simulink model "MATMPC_SIMULINK_R2022b"  (R2022b)
settings: Solver=ode4  StartTime=0.0  StopTime=10  RelTol=1e-3
values from neighbouring files (symbols this model uses):
  lb = 0    [Initialization_Simulink.m]
  lbu = -inf(nu,1)    [InitData.m]    (also in Initialization_Simulink.m = repmat(lbu,1,N))
  lbx = 0    [Initialization_Simulink.m]
  para = repmat(para0,1,N+1)    [InitData.m]    (also in Initialization_Simulink.m)
  Ts = settings.Ts_st    [Initialization_Simulink.m]    (also in Simulation.m)
  ub = 0    [Initialization_Simulink.m]
  ubu = inf(nu,1)    [InitData.m]    (also in Initialization_Simulink.m = repmat(ubu,1,N))
  ubx = 0    [Initialization_Simulink.m]
  W = repmat([Qp Qrpy Qq Qv Qomega Qdu]',1,N)    [Initialization_Simulink.m]
  WN = [Qp Qrpy Qq Qv Qomega]'    [Initialization_Simulink.m]
  x0 = [ ... (first row only)    [Initialization_Simulink.m]
  z0 = 0    [Initialization_Simulink.m]
undefined symbols (not defined in the file or in its folder): opt, settings
libraries: sharedtransform x1, simulink_extras x1, sharedTrackingLibrary x1
settings Model: Creator=chen  LastModifiedBy=beniamino
settings SolverCC: AlgebraicLoopSolver=TrustRegion
settings DataIOCC: ReturnWorkspaceOutputs=off
settings DebuggingCC: UnconnectedInputMsg=warning  UnconnectedOutputMsg=warning  UnconnectedLineMsg=warning  SFMachineParentedDataDiag=warning  ArithmeticOperatorsInVariantConditions=warning
settings ModelReferenceCC: EnableRefExpFcnMdlSchedulingChecks=on
settings SFSimCC: SimUseLocalCustomCode=off  CustomCodeUndefinedFunction=UseInterfaceOnly
settings RTWCC: RTWUseLocalCustomCode=off  CheckMdlBeforeBuild=Error

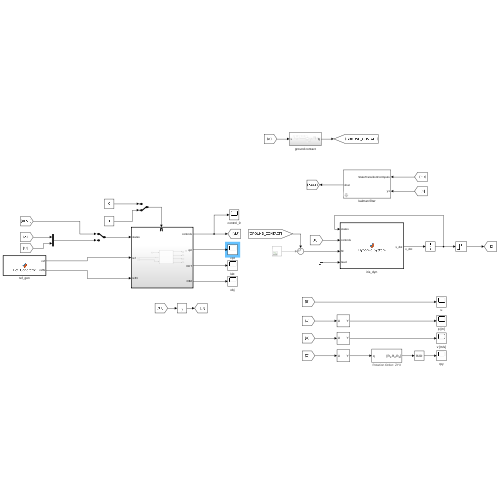
[thumbnail: Simulink's stored preview of the top-level diagram]
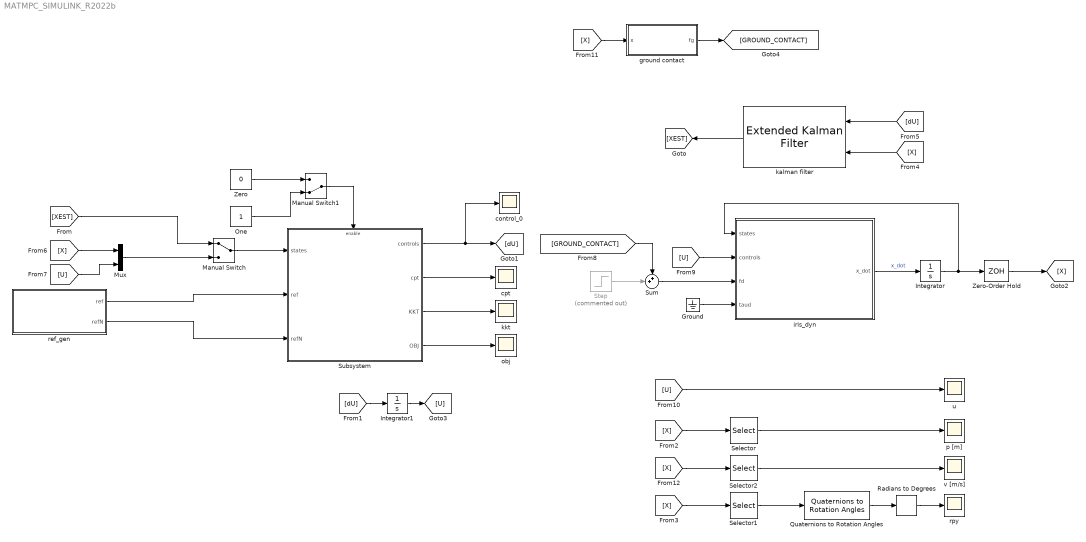
== system MATMPC_SIMULINK_R2022b ==
  Ground : Ground
  Integrator : Integrator  InitialCondition=x0(1:13)
  Integrator1 : Integrator  InitialCondition=[0.5 0.5 0.5 0.5]
  Manual Switch : ManualSwitch
  Manual Switch1 : ManualSwitch  CurrentSetting=0
  Mux : Mux  Inputs=2
  One : Constant  OutDataTypeStr=Inherit: Inherit via back propagation
  Quaternions to Rotation Angles : sharedtransform/Quaternions to Rotation Angles  rotationOrder=ZYX  aMode=aMode
  Radians to Degrees : simulink_extras/Transformations/Radians to Degrees
  Selector : Selector  InputPortWidth=13  IndexOptions=Index vector (dialog)  Indices=[1 2 3]  OutputSizes=1
  Selector1 : Selector  InputPortWidth=13  IndexOptions=Index vector (dialog)  Indices=4:7  OutputSizes=1
  Selector2 : Selector  InputPortWidth=13  IndexOptions=Index vector (dialog)  Indices=8:10  OutputSizes=1
  Step : Step  Commented=on  Time=5  Before=[0 0 0]  After=[1 0 0]  SampleTime=Ts
  Subsystem : Subsystem
  Sum : Sum  Inputs=++|
  Zero : Constant  Value=0  OutDataTypeStr=Inherit: Inherit via back propagation
  Zero-Order Hold : ZeroOrderHold  SampleTime=Ts
  control_0 : Scope
  cpt : Scope
  ground contact : Subsystem
  iris_dyn : MATLAB Function  TreatAsAtomicUnit=on
  kalman filter : sharedTrackingLibrary/Extended Kalman Filter  StateTransitionFcn=irisStateTransitionFcn  HasStateTransitionJacobianFcn=off  HasAdditiveProcessNoise=Additive  ProcessNoise=Q  HasTimeVaryingProcessNoise=off  HasStateTransitionFcnExtraArgument=1  InitialState=x0  InitialStateCovariance=Q0  MeasurementFcn1=irisMeasurementFcn  HasMeasurementJacobianFcn1=off  HasMeasurementEnablePort1=off  HasAdditiveMeasurementNoise1=Additive  MeasurementNoise1=R  HasTimeVaryingMeasurementNoise1=off  HasMeasurementFcnExtraArgument1=0  HasMeasurementWrapping1=off  MeasurementFcn2=myMeasurementFcn  HasMeasurementJacobianFcn2=off  HasMeasurementEnablePort2=off  HasAdditiveMeasurementNoise2=Additive  MeasurementNoise2=1  HasTimeVaryingMeasurementNoise2=off  HasMeasurementFcnExtraArgument2=0  HasMeasurementWrapping2=off  MeasurementFcn3=myMeasurementFcn  HasMeasurementJacobianFcn3=off  HasMeasurementEnablePort3=off  HasAdditiveMeasurementNoise3=Additive  MeasurementNoise3=1  HasTimeVaryingMeasurementNoise3=off  HasMeasurementFcnExtraArgument3=0  HasMeasurementWrapping3=off  MeasurementFcn4=myMeasurementFcn  HasMeasurementJacobianFcn4=off  HasMeasurementEnablePort4=off  HasAdditiveMeasurementNoise4=Additive  MeasurementNoise4=1  HasTimeVaryingMeasurementNoise4=off  HasMeasurementFcnExtraArgument4=0  HasMeasurementWrapping4=off  MeasurementFcn5=myMeasurementFcn  HasMeasurementJacobianFcn5=off  HasMeasurementEnablePort5=off  HasAdditiveMeasurementNoise5=Additive  MeasurementNoise5=1  HasTimeVaryingMeasurementNoise5=off  HasMeasurementFcnExtraArgument5=0  HasMeasurementWrapping5=off  EnableMultirate=off  StateTransitionFcnSampleTime=1  MeasurementFcn1SampleTime=1  MeasurementFcn2SampleTime=1  MeasurementFcn3SampleTime=1  MeasurementFcn4SampleTime=1  MeasurementFcn5SampleTime=1  UseCurrentEstimator=off  OutputStateCovariance=off  DataType=double  SampleTime=Ts  NumberOfMeasurements=1
  kkt : Scope
  obj : Scope
  p [m] : Scope
  ref_gen : MATLAB Function  TreatAsAtomicUnit=on
  rpy : Scope
  u : Scope
  v [m/s] : Scope
  wires:
  iris_dyn/1(x_dot) -> Integrator/1  "x_dot"
  Selector/1 -> p [m]/1
  Selector1/1 -> Quaternions to Rotation Angles/1
  Quaternions to Rotation Angles/1 -> Radians to Degrees/1
  Radians to Degrees/1 -> rpy/1
  [XEST] -> Manual Switch/1
  [dU] -> Integrator1/1
  [U] -> iris_dyn/2(controls)
  [X] -> Selector/1
  [X] -> Selector1/1
  Zero-Order Hold/1 -> [X]
  [dU] -> kalman filter/1
  [X] -> kalman filter/2
  kalman filter/1 -> [XEST]
  Integrator/1 -> iris_dyn/1(states), Zero-Order Hold/1
  [U] -> Mux/2
  [X] -> Mux/1
  Mux/1 -> Manual Switch/2
  Integrator1/1 -> [U]
  [U] -> u/1
  Ground/1 -> iris_dyn/4(taud)
  Step/1 -> Sum/2
  Sum/1 -> iris_dyn/3(fd)
  [GROUND_CONTACT] -> Sum/1
  [X] -> ground contact/1(x)
  ground contact/1(fg) -> [GROUND_CONTACT]
  Subsystem/1(controls) -> [dU], control_0/1
  Manual Switch/1 -> Subsystem/1(states)
  ref_gen/1(ref) -> Subsystem/2(ref)
  ref_gen/2(refN) -> Subsystem/3(refN)
  Subsystem/2(cpt) -> cpt/1
  Subsystem/3(KKT) -> kkt/1
  Subsystem/4(OBJ) -> obj/1
  Manual Switch1/1 -> Subsystem/Enable
  Zero/1 -> Manual Switch1/1
  One/1 -> Manual Switch1/2
  [X] -> Selector2/1
  Selector2/1 -> v [m/s]/1

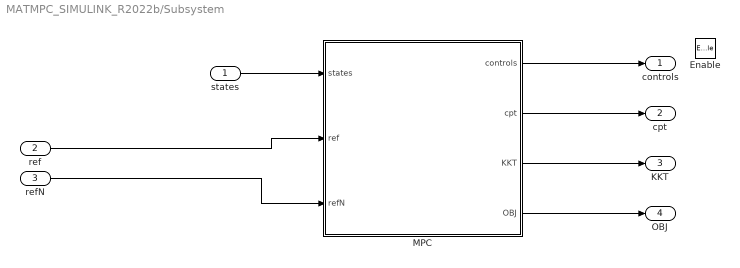
== system MATMPC_SIMULINK_R2022b/Subsystem ==
  states : Inport
  ref : Inport  Port=2
  refN : Inport  Port=3
  Enable : EnablePort
  MPC : MATLAB Function  TreatAsAtomicUnit=on  SystemSampleTime=Ts
  controls : Outport  OutputWhenDisabled=reset  InitialOutput=[0 0 0 0]
  cpt : Outport  Port=2
  KKT : Outport  Port=3
  OBJ : Outport  Port=4
  wires:
  MPC/2(cpt) -> cpt/1
  MPC/3(KKT) -> KKT/1
  MPC/4(OBJ) -> OBJ/1
  MPC/1(controls) -> controls/1
  refN/1 -> MPC/3(refN)
  ref/1 -> MPC/2(ref)
  states/1 -> MPC/1(states)

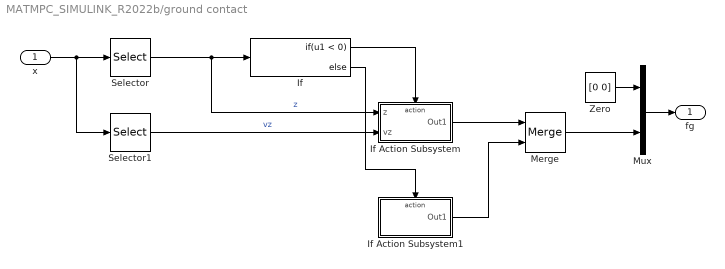
== system MATMPC_SIMULINK_R2022b/ground contact ==
  x : Inport
  If : If  IfExpression=u1 < 0
  If Action Subsystem : Subsystem  TreatAsAtomicUnit=on
  If Action Subsystem1 : Subsystem  TreatAsAtomicUnit=on
  Merge : Merge
  Mux : Mux  Inputs=2
  Selector : Selector  InputPortWidth=13  IndexOptions=Index vector (dialog)  Indices=3  OutputSizes=1
  Selector1 : Selector  InputPortWidth=13  IndexOptions=Index vector (dialog)  Indices=10  OutputSizes=1
  Zero : Constant  Value=[0 0]  OutDataTypeStr=Inherit: Inherit via back propagation
  fg : Outport
  wires:
  x/1 -> Selector1/1, Selector/1
  Mux/1 -> fg/1
  Zero/1 -> Mux/1
  Merge/1 -> Mux/2
  Selector/1 -> If Action Subsystem/1(z), If/1  "z"
  If/1 -> If Action Subsystem/Action
  If Action Subsystem/1(Out1) -> Merge/1
  If/2 -> If Action Subsystem1/Action
  If Action Subsystem1/1(Out1) -> Merge/2
  Selector1/1 -> If Action Subsystem/2(vz)  "vz"

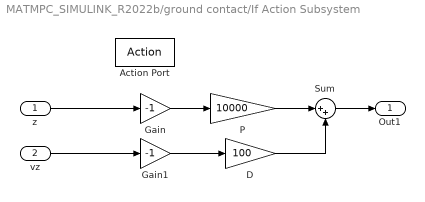
== system MATMPC_SIMULINK_R2022b/ground contact/If Action Subsystem ==
  z : Inport
  vz : Inport  Port=2
  Action Port : ActionPort  ActionPortLabel=if(u1 < 0)
  D : Gain  Gain=100
  Gain : Gain  Gain=-1
  Gain1 : Gain  Gain=-1
  P : Gain  Gain=10000
  Sum : Sum  Inputs=|++
  Out1 : Outport
  wires:
  z/1 -> Gain/1
  Gain/1 -> P/1
  P/1 -> Sum/1
  Sum/1 -> Out1/1
  D/1 -> Sum/2
  vz/1 -> Gain1/1
  Gain1/1 -> D/1

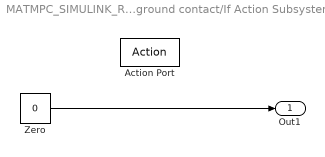
== system MATMPC_SIMULINK_R2022b/ground contact/If Action Subsystem1 ==
  Action Port : ActionPort  ActionPortLabel=else
  Zero : Constant  Value=0  OutDataTypeStr=Inherit: Inherit via back propagation
  Out1 : Outport
  wires:
  Zero/1 -> Out1/1

== matlab function MATMPC_SIMULINK_R2022b/ref_gen ==
  data: ref output; settings parameter; refN output
function [ref,refN] = Ref_Generator(settings)

p_ref = [0 0 30];
rpy_ref = [0 0 0];
q_ref = [1 0 0 0];
v_ref = [0 0 0];
omega_ref = [0 0 0];
du_ref = zeros(1,4);
t_ref = [p_ref rpy_ref q_ref v_ref omega_ref du_ref];
t_refN = t_ref(1:settings.nyN);

ref = repmat(t_ref',1,settings.N);
refN = t_refN';

%ref=zeros(settings.ny,settings.N);
%refN=zeros(settings.nyN,1);

%     ref = repmat([1.4, 0, 0]',1,settings.N);
%     refN = 1.4;

== matlab function MATMPC_SIMULINK_R2022b/iris_dyn ==
  data: states input size=nx-4; x_dot output size=nx-4; controls input size=nu; fd input size=3; taud input size=3
function x_dot  = Dynamic_System(states,controls, fd, taud)

g = 9.81; % gravity [m/s^2]

mR = 1.5; % drone mass [Kg]
JR = 0.15; % drone inertia
c_t_raw = 5.84e-06; % thrust coefficient [N/s^2]
c_tau_raw = c_t_raw * 0.06; % drag coefficient [Nm/s^2]
rotor_max_vel = 1100; % [rad/s]
c_direction = [-1 -1 1 1]; % 1: CW , -1: CCW
p_mot = ... % rotor position in body frame [m]
    [0.13 -0.22 0;
    -0.13 0.2 0;
    0.13 0.22 0;
    -0.13 -0.2 0];
theta = atan2(p_mot(:,2),p_mot(:,1)); % arm direction angle
l = vecnorm(p_mot,2,2); % arm length

c_t = c_t_raw .* rotor_max_vel.^2;
c_tau = c_tau_raw .* rotor_max_vel.^2;

p=states(1:3);
q=states(4:7);
v=states(8:10);
omega=states(11:13);
u=controls(1:4); % propeller angular rate square

% quaternion conversions
eta = q(1);
epsilon = q(2:4);
epsilon_x = [0, -epsilon(3), epsilon(2); epsilon(3), 0, -epsilon(1); -epsilon(2), epsilon(1), 0]; 
Rq = eye(3) + 2*eta*epsilon_x + 2*epsilon_x^2;
Mq = [eta, -epsilon'; epsilon, eta*eye(3)+epsilon_x];

% thrust matrix

F_temp = [...
    0, 0, 0, 0;...
    0, 0, 0, 0;...
    1, 1, 1, 1];
F = 1/mR .* c_t .* F_temp;

% torque matrix
M = c_tau .* F_temp * diag(c_direction) + ...
    c_t .* [...
    sin(theta(1)), sin(theta(2)), sin(theta(3)), sin(theta(4));...
    -cos(theta(1)), -cos(theta(2)), -cos(theta(3)), -cos(theta(4));...
    0, 0, 0, 0]...
    *diag(l);


% explicit ODE RHS
x_dot = [
    v
    1/2*Mq*[0;omega]
    Rq*F*u - [0;0;g] + 1/mR*fd
    1/JR.* M*u + 1/JR*taud
    ];

return

== matlab function MATMPC_SIMULINK_R2022b/Subsystem/MPC ==
  settings: updateMethod=DISCRETE  sampleTime=0.01
  data: states input size=nx; settings parameter; opt parameter; lb parameter; ub parameter; lbx parameter; ubx parameter; lbu parameter; ubu parameter; W parameter; WN parameter; para parameter; ref input size=[ny N]; refN input size=nyN; z0 parameter; controls output size=nu; cpt output size=1; KKT output; OBJ output
function [controls, cpt, KKT, OBJ] = NMPC_BLOCK(states, settings, opt, lb, ub, lbx, ubx, lbu, ubu, W, WN, para, ref, refN, z0)

%% everything should has a fixed size
coder.extrinsic('mpc_nmpcsolver_simulink');  
coder.extrinsic('InitData');  
coder.extrinsic('InitMemory');  
coder.extrinsic('evalin');
coder.extrinsic('assignin');

%%

persistent x u z lambda mu mu_x mu_u;
persistent input mem;

if isempty(input)  
    
    nx = settings.nx;        % No. of differential states
    nu = settings.nu;        % No. of controls
    nz = settings.nz;        % No. of algebraic states
    ny = settings.ny;        % No. of outputs (references)    
    nyN= settings.nyN;       % No. of outputs at terminal stage 
    np = settings.np;        % No. of parameters (on-line data)
    nc = settings.nc;        % No. of constraints
    ncN = settings.ncN;      % No. of constraints at terminal stage
    nbu = settings.nbu;      % No. of control bounds
    nbx = settings.nbx;      % No. of state bounds
    nbu_idx = settings.nbu_idx; % Index of control bounds
    nbx_idx = settings.nbx_idx; % Index of state bounds
    N = settings.N;
    N2 = settings.N2;
    r = settings.r;
        
    input.x0=states;
    
    x=repmat(states,1,N+1);
    input.x=x;
    
    u=zeros(nu,N);
    input.u=u;
    
    z=repmat(z0,1,N);
    input.z=z;
    
    lambda = zeros(nx,N+1);
    input.lambda= lambda;
    
    if N*nc+ncN > 0
        mu = zeros(N*nc+ncN,1);
    else
        mu = 0;
    end
    input.mu= mu;
    
    mu_u = zeros(N*nu,1);
    input.mu_u= mu_u;
    
    if N*nbx > 0
        mu_x = zeros(N*nbx,1);
    else
        mu_x = 0;
    end
    input.mu_x = mu_x;
    
    input.W=W;
    input.WN=WN;
    input.od = para;
    
    input.lb = lb;
    input.ub = ub;
    input.lbx = lbx;
    input.ubx = ubx;
    input.lbu = lbu;
    input.ubu = ubu;
      
    input.y = ref;
    input.yN = refN;
    
    mem = InitMemory(settings, opt, input);
        
else

    input.x=x; 
    input.u=u;
    input.z=z;
    input.lambda=lambda;   
    input.mu=mu;
    input.mu_x=mu_x;
    input.mu_u=mu_u;
    
end

%%
cpt = 0;
KKT = 0;
OBJ = 0;
input.x0 = states;
[input,mem,cpt,KKT,OBJ] = mpc_nmpcsolver_simulink(input, settings, mem, opt);
controls = input.u(:,1);

%% shifting
switch opt.shifting
    case 'yes'
        x=[input.x(:,2:end),input.x(:,end)];  
        u=[input.u(:,2:end),input.u(:,end)]; 
        z=[input.z(:,2:end),input.z(:,end)]; 
        lambda=[input.lambda(:,2:end),input.lambda(:,end)];
        if (settings.N*settings.nc+settings.ncN) >0
            mu(1:end-settings.ncN+1)=input.mu(settings.nc+1:settings.N*settings.nc+settings.ncN,1);
            mu(settings.N*settings.nc+1:end)=input.mu(settings.N*settings.nc+settings.ncN-settings.nc+1:settings.N*settings.nc+settings.ncN,1);
        else
            mu=0;
        end
        mu_x=[input.mu_x(2:end,1);input.mu_x(end,1)];
        mu_u=[input.mu_u(2:end,1);input.mu_u(end,1)];
   case 'no'
        x=input.x;
        u=input.u;
        z=input.z;
        lambda=input.lambda;
        mu=input.mu;
        mu_x=input.mu_x;
        mu_u=input.mu_u;
end

return
